simulink model "hyd_hyb_2_int_cont_Final_AMT"  (R2013b)
settings: Solver=ode4  StartTime=0  StopTime=3005  FixedStep=0.01  MaxStep=.4  RelTol=1e-8
InitFcn:
  | const_3_new
values from neighbouring files (symbols this model uses):
  Af = 6.3    [brk_enrg.m]    (also in brk_enrg_1.m)
  BSFC_906_205 = [3.5684 4.3466 5.1668 6.0769 6.988 7.8992 8.8104 9.7336 10.8548 11.9809 13.1112 14.2571 ... (663 elements, 39x17)]    [BSFC_map_906_205.mat]
  Cd = 0.55    [brk_enrg.m]    (also in brk_enrg_1.m)
  den = 1.202    [brk_enrg.m]    (also in brk_enrg_1.m)
  fr = 0.01    [brk_enrg.m]    (also in brk_enrg_1.m)
undefined symbols (not defined in the file or in its folder): clutchRise, down_spd_2, down_spd_3, down_spd_4, down_spd_c, Driving_Cycle, fuel_density, gearshift, I_wheel, Idle_spd_eng_906, M1_hydr, p_v_15, pmax_125, qv_125, Rw, sec_eng_sfc_map, T0, T1, T_max_906, T_min, TC_spd_ratio_max, teta_new_10, torque_convertor, Twait, up_spd_1, up_spd_2, up_spd_3, up_spd_c, v_p_10, v_p_15, v_p_5
libraries: neural x1742, fl_lib x43, nesl_utility x30, sdl_lib x14, simulink x4, simulink_need_slupdate x1
(part 13 of 26)

== system hyd_hyb_2_int_cont_Final_AMT/controller1/optimized controller/SOC upper 0.5/SOC under 0.6/net_loc_rod_5_6/Layer 3/Delays 1 ==
  "p{3}" : Inport  PortDimensions=60
  mux : Mux  Inputs=1
  "pd{3,2}" : Outport
  wires:
  "p{3}"/1 -> mux/1
  mux/1 -> "pd{3,2}"/1

== system hyd_hyb_2_int_cont_Final_AMT/controller1/optimized controller/SOC upper 0.5/SOC under 0.6/net_loc_rod_5_6/Layer 3/LW{3,2} ==
  "ad{3,2}" : Inport  PortDimensions=60
  "IW{3,2}(1,:)'" : Constant  Value=[0.21278300477895107;0.51344852513289463;-0.037590241773840127;0.87426964561402842;0.47883974451806377;-0.50784781099782816;-0.42443313454818898;-0.63652603538509656;0.70423364527984744;0.58568292864178184;-0.52796615746288977;-0.44287483766577246;0.86901354772123618;-0.13831685526252785;0.86566149289060479;0.64403142490178156;0.71733541437838555;0.027462260085903828;-0.37265143230844694;0.71199097292665836;-1.0092668976607591;0.54326870405319294;-0.22161113024701684;0.22850993838939238;-0.056916095287317267;-0.91628445056316477;-0.91086476780370962;-0.060619157895533675;0.93064231354933902;0.57914173943359415;0.22128542734464982;0.7199158978518877;0.9270211186610392;-0.82882792624492585;-0.35445656093166766;0.56586404922693345;0.21840031287896147;0.12031889714860289;0.61358543472489502;-0.34437004445453206;-0.49319773551856233;0.74417786809055086;0.83416465722893218;0.025074562352173025;-0.65605871255971948;-0.98066330920260369;-0.79678322946662417;-0.33944765090641305;-0.80799595485443365;0.73951954905542505;0.90293635064930589;-0.53403515470352247;-0.99336400775468636;0.86698814398730517;-0.5677534071583421;-0.32793471469176605;0.14570127648050649;0.0087963951498697922;-0.6729797739571125;0.31101959537299745]
  Mux : Mux  Inputs=1
  dotprod1 : neural/Weight Functions/dotprod
  "lz{3,2}" : Outport
  wires:
  "IW{3,2}(1,:)'"/1 -> dotprod1/1
  "ad{3,2}"/1 -> dotprod1/2
  dotprod1/1 -> Mux/1
  Mux/1 -> "lz{3,2}"/1

== system hyd_hyb_2_int_cont_Final_AMT/controller1/optimized controller/SOC upper 0.5/SOC upper 0.6/SOC under 0.7/net_col_a_b_6_1/Layer 1 ==
  "p{1}" : Inport  PortDimensions=2
  Delays 1 : Subsystem
  "IW{1,1}" : Subsystem
  "b{1}" : Constant  Value=[5.4291259813067461;4.718478314630234;3.7592821803800116;-3.1787920472608406;2.2590998726780076;1.3899147707624782;0.87327049833135528;-0.021254336575357417;-0.80530109394321947;-1.4715401148994816;2.2200413751043135;3.0289705769041251;3.923020910366191;4.6547090616272833;5.4114556646704166]
  netsum : Sum  Inputs=2  SaturateOnIntegerOverflow=on  InputSameDT=on  OutDataTypeStr=Inherit: Same as first input
  tansig : neural/Transfer Functions/tansig
  "a{1}" : Outport  InitialOutput=[0;0;0;0;0;0;0;0;0;0;0;0;0;0;0]
  wires:
  "p{1}"/1 -> Delays 1/1("p{1}")
  Delays 1/1("pd{1,1}") -> "IW{1,1}"/1("pd{1,1}")
  "IW{1,1}"/1("iz{1,1}") -> netsum/1
  "b{1}"/1 -> netsum/2
  netsum/1 -> tansig/1
  tansig/1 -> "a{1}"/1

== system hyd_hyb_2_int_cont_Final_AMT/controller1/optimized controller/SOC upper 0.5/SOC upper 0.6/SOC under 0.7/net_col_a_b_6_1/Layer 2 ==
  "a{1} " : Inport  PortDimensions=15
  Delays 1 : Subsystem
  "LW{2,1}" : Subsystem
  "b{2}" : Constant  Value=[-1.646349611515898;-1.5096703195224832;1.3949167909537323;1.1533080996131411;0.98809756853578845;-0.68129902029256906;0.56728877028882763;0.46578866737002761;-0.33256964616945445;0.14197265823532756;-0.011470087521661837;0.27403951081779188;0.44394331190764186;0.63896055064956137;0.67829391232291314;0.97113533342800851;-1.1922907318745983;1.2971020916511706;1.529818326598521;1.6930343749454633]
  netsum : Sum  Inputs=2  SaturateOnIntegerOverflow=on  InputSameDT=on  OutDataTypeStr=Inherit: Same as first input
  tansig : neural/Transfer Functions/tansig
  "a{2}" : Outport  InitialOutput=[0;0;0;0;0;0;0;0;0;0;0;0;0;0;0;0;0;0;0;0]
  wires:
  "a{1} "/1 -> Delays 1/1("p{2}")
  Delays 1/1("pd{2,1}") -> "LW{2,1}"/1("ad{2,1}")
  "LW{2,1}"/1("lz{2,1}") -> netsum/1
  "b{2}"/1 -> netsum/2
  netsum/1 -> tansig/1
  tansig/1 -> "a{2}"/1

== system hyd_hyb_2_int_cont_Final_AMT/controller1/optimized controller/SOC upper 0.5/SOC upper 0.6/SOC under 0.7/net_col_a_b_6_1/Layer 3 ==
  "a{2} " : Inport  PortDimensions=20
  Delays 1 : Subsystem
  "LW{3,2}" : Subsystem
  "b{3}" : Constant  Value=0.042619569041635712
  netsum : Sum  Inputs=2  SaturateOnIntegerOverflow=on  InputSameDT=on  OutDataTypeStr=Inherit: Same as first input
  purelin : neural/Transfer Functions/purelin
  "a{3}" : Outport  InitialOutput=0
  wires:
  "a{2} "/1 -> Delays 1/1("p{3}")
  Delays 1/1("pd{3,2}") -> "LW{3,2}"/1("ad{3,2}")
  "LW{3,2}"/1("lz{3,2}") -> netsum/1
  "b{3}"/1 -> netsum/2
  netsum/1 -> purelin/1
  purelin/1 -> "a{3}"/1

== system hyd_hyb_2_int_cont_Final_AMT/controller1/optimized controller/SOC upper 0.5/SOC upper 0.6/SOC under 0.7/net_col_a_b_6_1/Process Input 1 ==
  x : Inport  PortDimensions=2
  fixunknowns : neural/Processing Functions/fixunknowns  inputSize=2  indices=[1 2]
  mapminmax : neural/Processing Functions/mapminmax  xmin=[0.011694642437567444;0.050000000000000003]  xmax=[1;0.94394666666666693]  ymin=-1  ymax=1
  removeconstantrows : neural/Processing Functions/removeconstantrows  inputSize=2  keep=[1 2]
  p : Outport  PortDimensions=2
  wires:
  x/1 -> fixunknowns/1
  fixunknowns/1 -> removeconstantrows/1
  removeconstantrows/1 -> mapminmax/1
  mapminmax/1 -> p/1

== system hyd_hyb_2_int_cont_Final_AMT/controller1/optimized controller/SOC upper 0.5/SOC upper 0.6/SOC under 0.7/net_col_a_b_6_1/Process Output 1 ==
  a : Inport  PortDimensions=1
  mapminmax_reverse : neural/Processing Functions/mapminmax_reverse  xmin=0  xmax=1  ymin=-1  ymax=1
  removeconstantrows_reverse : neural/Processing Functions/removeconstantrows_reverse  inputSize=1  constants=zeros(0,1)  rearrange=1
  y : Outport  PortDimensions=1
  wires:
  a/1 -> mapminmax_reverse/1
  mapminmax_reverse/1 -> removeconstantrows_reverse/1
  removeconstantrows_reverse/1 -> y/1

== system hyd_hyb_2_int_cont_Final_AMT/controller1/optimized controller/SOC upper 0.5/SOC upper 0.6/SOC under 0.7/net_col_a_b_6_7/Layer 1 ==
  "p{1}" : Inport  PortDimensions=2
  Delays 1 : Subsystem
  "IW{1,1}" : Subsystem
  "b{1}" : Constant  Value=[5.4291259813067461;4.718478314630234;3.7592821803800116;-3.1787920472608406;2.2590998726780076;1.3899147707624782;0.87327049833135528;-0.021254336575357417;-0.80530109394321947;-1.4715401148994816;2.2200413751043135;3.0289705769041251;3.923020910366191;4.6547090616272833;5.4114556646704166]
  netsum : Sum  Inputs=2  SaturateOnIntegerOverflow=on  InputSameDT=on  OutDataTypeStr=Inherit: Same as first input
  tansig : neural/Transfer Functions/tansig
  "a{1}" : Outport  InitialOutput=[0;0;0;0;0;0;0;0;0;0;0;0;0;0;0]
  wires:
  tansig/1 -> "a{1}"/1
  netsum/1 -> tansig/1
  "b{1}"/1 -> netsum/2
  "IW{1,1}"/1("iz{1,1}") -> netsum/1
  Delays 1/1("pd{1,1}") -> "IW{1,1}"/1("pd{1,1}")
  "p{1}"/1 -> Delays 1/1("p{1}")

== system hyd_hyb_2_int_cont_Final_AMT/controller1/optimized controller/SOC upper 0.5/SOC upper 0.6/SOC under 0.7/net_col_a_b_6_7/Layer 2 ==
  "a{1} " : Inport  PortDimensions=15
  Delays 1 : Subsystem
  "LW{2,1}" : Subsystem
  "b{2}" : Constant  Value=[-1.646349611515898;-1.5096703195224832;1.3949167909537323;1.1533080996131411;0.98809756853578845;-0.68129902029256906;0.56728877028882763;0.46578866737002761;-0.33256964616945445;0.14197265823532756;-0.011470087521661837;0.27403951081779188;0.44394331190764186;0.63896055064956137;0.67829391232291314;0.97113533342800851;-1.1922907318745983;1.2971020916511706;1.529818326598521;1.6930343749454633]
  netsum : Sum  Inputs=2  SaturateOnIntegerOverflow=on  InputSameDT=on  OutDataTypeStr=Inherit: Same as first input
  tansig : neural/Transfer Functions/tansig
  "a{2}" : Outport  InitialOutput=[0;0;0;0;0;0;0;0;0;0;0;0;0;0;0;0;0;0;0;0]
  wires:
  tansig/1 -> "a{2}"/1
  netsum/1 -> tansig/1
  "b{2}"/1 -> netsum/2
  "LW{2,1}"/1("lz{2,1}") -> netsum/1
  Delays 1/1("pd{2,1}") -> "LW{2,1}"/1("ad{2,1}")
  "a{1} "/1 -> Delays 1/1("p{2}")

== system hyd_hyb_2_int_cont_Final_AMT/controller1/optimized controller/SOC upper 0.5/SOC upper 0.6/SOC under 0.7/net_col_a_b_6_7/Layer 3 ==
  "a{2} " : Inport  PortDimensions=20
  Delays 1 : Subsystem
  "LW{3,2}" : Subsystem
  "b{3}" : Constant  Value=0.042619569041635712
  netsum : Sum  Inputs=2  SaturateOnIntegerOverflow=on  InputSameDT=on  OutDataTypeStr=Inherit: Same as first input
  purelin : neural/Transfer Functions/purelin
  "a{3}" : Outport  InitialOutput=0
  wires:
  purelin/1 -> "a{3}"/1
  netsum/1 -> purelin/1
  "b{3}"/1 -> netsum/2
  "LW{3,2}"/1("lz{3,2}") -> netsum/1
  Delays 1/1("pd{3,2}") -> "LW{3,2}"/1("ad{3,2}")
  "a{2} "/1 -> Delays 1/1("p{3}")

== system hyd_hyb_2_int_cont_Final_AMT/controller1/optimized controller/SOC upper 0.5/SOC upper 0.6/SOC under 0.7/net_col_a_b_6_7/Process Input 1 ==
  x : Inport  PortDimensions=2
  fixunknowns : neural/Processing Functions/fixunknowns  inputSize=2  indices=[1 2]
  mapminmax : neural/Processing Functions/mapminmax  xmin=[0.011694642437567444;0.050000000000000003]  xmax=[1;0.94394666666666693]  ymin=-1  ymax=1
  removeconstantrows : neural/Processing Functions/removeconstantrows  inputSize=2  keep=[1 2]
  p : Outport  PortDimensions=2
  wires:
  mapminmax/1 -> p/1
  removeconstantrows/1 -> mapminmax/1
  fixunknowns/1 -> removeconstantrows/1
  x/1 -> fixunknowns/1

== system hyd_hyb_2_int_cont_Final_AMT/controller1/optimized controller/SOC upper 0.5/SOC upper 0.6/SOC under 0.7/net_col_a_b_6_7/Process Output 1 ==
  a : Inport  PortDimensions=1
  mapminmax_reverse : neural/Processing Functions/mapminmax_reverse  xmin=0  xmax=1  ymin=-1  ymax=1
  removeconstantrows_reverse : neural/Processing Functions/removeconstantrows_reverse  inputSize=1  constants=zeros(0,1)  rearrange=1
  y : Outport  PortDimensions=1
  wires:
  removeconstantrows_reverse/1 -> y/1
  mapminmax_reverse/1 -> removeconstantrows_reverse/1
  a/1 -> mapminmax_reverse/1

== system hyd_hyb_2_int_cont_Final_AMT/controller1/optimized controller/SOC upper 0.5/SOC upper 0.6/SOC under 0.7/net_col_e_f_6_7/Layer 1 ==
  "p{1}" : Inport  PortDimensions=2
  Delays 1 : Subsystem
  "IW{1,1}" : Subsystem
  "b{1}" : Constant  Value=[-8.8578922704763041;8.4042892360625192;-7.9500084893405489;7.492292740917911;-7.075297682831537;6.5653391411727364;6.140320418383804;-5.6306218037143498;5.2017310942740975;4.7779398662401924;-4.3096479437985149;-3.8694939533350459;-3.4026972434889582;2.9180363550485859;2.5233555299387724;2.0614869063433754;1.5965524496681351;-1.1423406487569012;0.64405884107426203;0.23295690475029907;0.21904951735863054;0.68273518079764783;1.1340220880771177;1.4628899047128925;-2.0189679486955385;-2.6776183293763673;2.9490574244714782;3.4373185112780584;3.8603599158778059;4.3183089131402985;-4.7896523588348439;5.2017411095223869;-5.6883600090125501;-6.1259092722430823;6.6028020849475491;7.0422452842927754;-7.4915663488509772;7.9665515781619485;-8.3941668997364953;-8.8548095629012451]
  netsum : Sum  Inputs=2  SaturateOnIntegerOverflow=on  InputSameDT=on  OutDataTypeStr=Inherit: Same as first input
  tansig : neural/Transfer Functions/tansig
  "a{1}" : Outport  InitialOutput=[0;0;0;0;0;0;0;0;0;0;0;0;0;0;0;0;0;0;0;0;0;0;0;0;0;0;0;0;0;0;0;0;0;0;0;0;0;0;0;0]
  wires:
  tansig/1 -> "a{1}"/1
  netsum/1 -> tansig/1
  "b{1}"/1 -> netsum/2
  "IW{1,1}"/1("iz{1,1}") -> netsum/1
  Delays 1/1("pd{1,1}") -> "IW{1,1}"/1("pd{1,1}")
  "p{1}"/1 -> Delays 1/1("p{1}")

== system hyd_hyb_2_int_cont_Final_AMT/controller1/optimized controller/SOC upper 0.5/SOC upper 0.6/SOC under 0.7/net_col_e_f_6_7/Layer 2 ==
  "a{1} " : Inport  PortDimensions=40
  Delays 1 : Subsystem
  "LW{2,1}" : Subsystem
  "b{2}" : Constant  Value=[-1.5481410379896341;-1.4722157754701299;-1.4182962377280097;-1.3387311384343061;1.2983921636824405;-1.210024697487539;1.1647052885200337;1.085322627026474;-1.0583259785438344;-1.0125038796374846;-0.92816237918533084;-0.84166214172462495;0.7720476266891465;-0.68862710060922727;-0.66180234799140847;0.55778737249163612;-0.5739733374634064;-0.45525711092005827;-0.40942953136334892;0.36574767859724377;0.27529894302507696;0.24383222824829606;0.19268525262761244;-0.0869252647609811;-0.040403947124311022;-0.031888545879754718;-0.05798707962786407;0.13694331166074308;0.24631659120042129;0.26591880237517995;0.32068778652282787;0.37526588045543213;-0.47498839316153901;0.51137673885021073;-0.5990164565810322;0.67203954642275587;0.7511674885213897;-0.77140397482380441;0.85976576557099027;-0.92388442298986573;0.96930527326269178;-1.0298098139986036;-1.1007021830056818;1.1648435654146696;1.2287555475076584;-1.2833186739340898;-1.3606363399356558;1.4167612982858691;-1.5157208154592794;1.5087905241510864]
  netsum : Sum  Inputs=2  SaturateOnIntegerOverflow=on  InputSameDT=on  OutDataTypeStr=Inherit: Same as first input
  tansig : neural/Transfer Functions/tansig
  "a{2}" : Outport  InitialOutput=[0;0;0;0;0;0;0;0;0;0;0;0;0;0;0;0;0;0;0;0;0;0;0;0;0;0;0;0;0;0;0;0;0;0;0;0;0;0;0;0;0;0;0;0;0;0;0;0;0;0]
  wires:
  tansig/1 -> "a{2}"/1
  netsum/1 -> tansig/1
  "b{2}"/1 -> netsum/2
  "LW{2,1}"/1("lz{2,1}") -> netsum/1
  Delays 1/1("pd{2,1}") -> "LW{2,1}"/1("ad{2,1}")
  "a{1} "/1 -> Delays 1/1("p{2}")

== system hyd_hyb_2_int_cont_Final_AMT/controller1/optimized controller/SOC upper 0.5/SOC upper 0.6/SOC under 0.7/net_col_e_f_6_7/Layer 3 ==
  "a{2} " : Inport  PortDimensions=50
  Delays 1 : Subsystem
  "LW{3,2}" : Subsystem
  "b{3}" : Constant  Value=-0.11506746394677372
  netsum : Sum  Inputs=2  SaturateOnIntegerOverflow=on  InputSameDT=on  OutDataTypeStr=Inherit: Same as first input
  purelin : neural/Transfer Functions/purelin
  "a{3}" : Outport  InitialOutput=0
  wires:
  purelin/1 -> "a{3}"/1
  netsum/1 -> purelin/1
  "b{3}"/1 -> netsum/2
  "LW{3,2}"/1("lz{3,2}") -> netsum/1
  Delays 1/1("pd{3,2}") -> "LW{3,2}"/1("ad{3,2}")
  "a{2} "/1 -> Delays 1/1("p{3}")

== system hyd_hyb_2_int_cont_Final_AMT/controller1/optimized controller/SOC upper 0.5/SOC upper 0.6/SOC under 0.7/net_col_e_f_6_7/Process Input 1 ==
  x : Inport  PortDimensions=2
  fixunknowns : neural/Processing Functions/fixunknowns  inputSize=2  indices=[1 2]
  mapminmax : neural/Processing Functions/mapminmax  xmin=[0.0027835059349667611;0.021539146666666665]  xmax=[1.009090909090909;0.58889400000000003]  ymin=-1  ymax=1
  removeconstantrows : neural/Processing Functions/removeconstantrows  inputSize=2  keep=[1 2]
  p : Outport  PortDimensions=2
  wires:
  mapminmax/1 -> p/1
  removeconstantrows/1 -> mapminmax/1
  fixunknowns/1 -> removeconstantrows/1
  x/1 -> fixunknowns/1

== system hyd_hyb_2_int_cont_Final_AMT/controller1/optimized controller/SOC upper 0.5/SOC upper 0.6/SOC under 0.7/net_col_e_f_6_7/Process Output 1 ==
  a : Inport  PortDimensions=1
  mapminmax_reverse : neural/Processing Functions/mapminmax_reverse  xmin=0  xmax=1  ymin=-1  ymax=1
  removeconstantrows_reverse : neural/Processing Functions/removeconstantrows_reverse  inputSize=1  constants=zeros(0,1)  rearrange=1
  y : Outport  PortDimensions=1
  wires:
  removeconstantrows_reverse/1 -> y/1
  mapminmax_reverse/1 -> removeconstantrows_reverse/1
  a/1 -> mapminmax_reverse/1

== system hyd_hyb_2_int_cont_Final_AMT/controller1/optimized controller/SOC upper 0.5/SOC upper 0.6/SOC under 0.7/net_loc_rod_6_7/Layer 1 ==
  "p{1}" : Inport  PortDimensions=2
  Delays 1 : Subsystem
  "IW{1,1}" : Subsystem
  "b{1}" : Constant  Value=[8.824474549246748;-8.3539581899361774;7.9180500965715499;7.4856270452295295;7.0291889559197109;-6.5160648504037608;-6.0051491737445231;-5.6799709048951863;5.19806155256191;4.7694002581991688;-4.2718293307910846;-3.7933727449376735;-3.4075974872825943;-2.9557662001981453;-2.4512826171554551;1.9968540619284594;-1.5180712033708814;-1.0823236947351929;0.65270333067677622;-0.22171360341636442;0.30648910984876571;-0.65165847547612499;-1.1471337479688715;1.5911971989977467;-2.0449450710405568;-2.4302538050746536;2.9621146231919044;-3.4741028886743219;3.8037991235467468;4.0802221372092466;-4.6712341146850189;-5.1980673102079908;5.6856540997831884;-6.1501781260260069;6.5094993739119937;-7.0017996579089372;-7.4043669072906422;7.8466649688215488;-8.274364497349513;8.7769344884722695]
  netsum : Sum  Inputs=2  SaturateOnIntegerOverflow=on  InputSameDT=on  OutDataTypeStr=Inherit: Same as first input
  tansig : neural/Transfer Functions/tansig
  "a{1}" : Outport  InitialOutput=[0;0;0;0;0;0;0;0;0;0;0;0;0;0;0;0;0;0;0;0;0;0;0;0;0;0;0;0;0;0;0;0;0;0;0;0;0;0;0;0]
  wires:
  tansig/1 -> "a{1}"/1
  netsum/1 -> tansig/1
  "b{1}"/1 -> netsum/2
  "IW{1,1}"/1("iz{1,1}") -> netsum/1
  Delays 1/1("pd{1,1}") -> "IW{1,1}"/1("pd{1,1}")
  "p{1}"/1 -> Delays 1/1("p{1}")

== system hyd_hyb_2_int_cont_Final_AMT/controller1/optimized controller/SOC upper 0.5/SOC upper 0.6/SOC under 0.7/net_loc_rod_6_7/Layer 2 ==
  "a{1} " : Inport  PortDimensions=40
  Delays 1 : Subsystem
  "LW{2,1}" : Subsystem
  "b{2}" : Constant  Value=[-1.5375109884301688;1.4171736518535769;1.52361155268007;1.3748031344760954;1.3228743192422741;1.2710869402908649;-1.2289478762921457;1.3043666245357657;1.1279084073962473;1.1592324888470029;1.0816615754733507;-1.1076579897629193;-0.91501169053418618;-0.94094658429811684;0.87746244560174713;0.94827946297111543;-0.85279014408642195;-0.55136865473041252;-0.71502898154289862;0.56062094302079912;-0.49981430410271727;0.5080931190367296;0.50678293785240025;-0.43330284501716315;0.24334211509970571;0.21958195465029282;-0.24935850636213924;-0.26038595402420367;0.19673396450795588;0.13998297555788999;-0.12995027624444025;0.073341413956929349;0.020500738682947012;0.10260269951590015;-0.011977356867705572;0.16529983194991943;0.27248116401324118;0.21972273308017506;0.27831436153061456;-0.37368385210235811;-0.35879821627249703;0.44905820177632477;0.4408842695857364;-0.52649284822534737;-0.52055294018007991;0.71915173123359;-0.57712246944047207;-0.639525224204745;0.78332227425292;-0.91876770100677474;0.74496747317097645;0.81162931619236156;-0.86905432344573885;0.94311832117696659;-1.052080950287456;-1.1540738973387714;1.1288625875898872;1.1443800540884874;1.2742597641129052;1.1542657972950399;-1.3842695887293082;1.4535463851249286;1.4217009587894542;-1.4529796844905569;-1.5186643879755066]
  netsum : Sum  Inputs=2  SaturateOnIntegerOverflow=on  InputSameDT=on  OutDataTypeStr=Inherit: Same as first input
  tansig : neural/Transfer Functions/tansig
  "a{2}" : Outport  InitialOutput=[0;0;0;0;0;0;0;0;0;0;0;0;0;0;0;0;0;0;0;0;0;0;0;0;0;0;0;0;0;0;0;0;0;0;0;0;0;0;0;0;0;0;0;0;0;0;0;0;0;0;0;0;0;0;0;0;0;0;0;0;0;0;0;0;0]
  wires:
  tansig/1 -> "a{2}"/1
  netsum/1 -> tansig/1
  "b{2}"/1 -> netsum/2
  "LW{2,1}"/1("lz{2,1}") -> netsum/1
  Delays 1/1("pd{2,1}") -> "LW{2,1}"/1("ad{2,1}")
  "a{1} "/1 -> Delays 1/1("p{2}")

== system hyd_hyb_2_int_cont_Final_AMT/controller1/optimized controller/SOC upper 0.5/SOC upper 0.6/SOC under 0.7/net_loc_rod_6_7/Layer 3 ==
  "a{2} " : Inport  PortDimensions=65
  Delays 1 : Subsystem
  "LW{3,2}" : Subsystem
  "b{3}" : Constant  Value=-0.44014037970907371
  netsum : Sum  Inputs=2  SaturateOnIntegerOverflow=on  InputSameDT=on  OutDataTypeStr=Inherit: Same as first input
  purelin : neural/Transfer Functions/purelin
  "a{3}" : Outport  InitialOutput=0
  wires:
  purelin/1 -> "a{3}"/1
  netsum/1 -> purelin/1
  "b{3}"/1 -> netsum/2
  "LW{3,2}"/1("lz{3,2}") -> netsum/1
  Delays 1/1("pd{3,2}") -> "LW{3,2}"/1("ad{3,2}")
  "a{2} "/1 -> Delays 1/1("p{3}")

== system hyd_hyb_2_int_cont_Final_AMT/controller1/optimized controller/SOC upper 0.5/SOC upper 0.6/SOC under 0.7/net_loc_rod_6_7/Process Input 1 ==
  x : Inport  PortDimensions=2
  fixunknowns : neural/Processing Functions/fixunknowns  inputSize=2  indices=[1 2]
  mapminmax : neural/Processing Functions/mapminmax  xmin=[0.0018488517726022993;0.17698999999999998]  xmax=[1;0.55617766666666668]  ymin=-1  ymax=1
  removeconstantrows : neural/Processing Functions/removeconstantrows  inputSize=2  keep=[1 2]
  p : Outport  PortDimensions=2
  wires:
  mapminmax/1 -> p/1
  removeconstantrows/1 -> mapminmax/1
  fixunknowns/1 -> removeconstantrows/1
  x/1 -> fixunknowns/1

== system hyd_hyb_2_int_cont_Final_AMT/controller1/optimized controller/SOC upper 0.5/SOC upper 0.6/SOC under 0.7/net_loc_rod_6_7/Process Output 1 ==
  a : Inport  PortDimensions=1
  mapminmax_reverse : neural/Processing Functions/mapminmax_reverse  xmin=0  xmax=1  ymin=-1  ymax=1
  removeconstantrows_reverse : neural/Processing Functions/removeconstantrows_reverse  inputSize=1  constants=zeros(0,1)  rearrange=1
  y : Outport  PortDimensions=1
  wires:
  removeconstantrows_reverse/1 -> y/1
  mapminmax_reverse/1 -> removeconstantrows_reverse/1
  a/1 -> mapminmax_reverse/1

== system hyd_hyb_2_int_cont_Final_AMT/controller1/optimized controller/SOC upper 0.5/SOC upper 0.6/SOC upper 0.7/SOC under 0.8/net_col_a_b_7_8 ==
  Input : Inport  PortDimensions=2
  Layer 1 : Subsystem
  Layer 2 : Subsystem
  Layer 3 : Subsystem
  Process Input 1 : Subsystem
  Process Output 1 : Subsystem
  Output : Outport  InitialOutput=0
  wires:
  Layer 3/1("a{3}") -> Process Output 1/1(a)
  [feedback2] -> Layer 3/1("a{2} ")
  Layer 2/1("a{2}") -> [feedback2]
  [feedback1] -> Layer 2/1("a{1} ")
  Layer 1/1("a{1}") -> [feedback1]
  Process Input 1/1(p) -> Layer 1/1("p{1}")
  Process Output 1/1(y) -> Output/1
  Input/1 -> Process Input 1/1(x)

== system hyd_hyb_2_int_cont_Final_AMT/controller1/optimized controller/SOC upper 0.5/SOC upper 0.6/SOC upper 0.7/SOC under 0.8/net_col_c_d_7_8 ==
  Input : Inport  PortDimensions=2
  Layer 1 : Subsystem
  Layer 2 : Subsystem
  Layer 3 : Subsystem
  Process Input 1 : Subsystem
  Process Output 1 : Subsystem
  Output : Outport  InitialOutput=0
  wires:
  Layer 3/1("a{3}") -> Process Output 1/1(a)
  [feedback2] -> Layer 3/1("a{2} ")
  Layer 2/1("a{2}") -> [feedback2]
  [feedback1] -> Layer 2/1("a{1} ")
  Layer 1/1("a{1}") -> [feedback1]
  Process Input 1/1(p) -> Layer 1/1("p{1}")
  Process Output 1/1(y) -> Output/1
  Input/1 -> Process Input 1/1(x)

== system hyd_hyb_2_int_cont_Final_AMT/controller1/optimized controller/SOC upper 0.5/SOC upper 0.6/SOC upper 0.7/SOC under 0.8/net_col_e_f_7_8 ==
  Input : Inport  PortDimensions=2
  Layer 1 : Subsystem
  Layer 2 : Subsystem
  Layer 3 : Subsystem
  Process Input 1 : Subsystem
  Process Output 1 : Subsystem
  Output : Outport  InitialOutput=0
  wires:
  Layer 3/1("a{3}") -> Process Output 1/1(a)
  [feedback2] -> Layer 3/1("a{2} ")
  Layer 2/1("a{2}") -> [feedback2]
  [feedback1] -> Layer 2/1("a{1} ")
  Layer 1/1("a{1}") -> [feedback1]
  Process Input 1/1(p) -> Layer 1/1("p{1}")
  Process Output 1/1(y) -> Output/1
  Input/1 -> Process Input 1/1(x)

== system hyd_hyb_2_int_cont_Final_AMT/controller1/optimized controller/SOC upper 0.5/SOC upper 0.6/SOC upper 0.7/SOC under 0.8/net_loc_rod_7_8 ==
  Input : Inport  PortDimensions=2
  Layer 1 : Subsystem
  Layer 2 : Subsystem
  Layer 3 : Subsystem
  Process Input 1 : Subsystem
  Process Output 1 : Subsystem
  Output : Outport  InitialOutput=0
  wires:
  Layer 3/1("a{3}") -> Process Output 1/1(a)
  [feedback2] -> Layer 3/1("a{2} ")
  Layer 2/1("a{2}") -> [feedback2]
  [feedback1] -> Layer 2/1("a{1} ")
  Layer 1/1("a{1}") -> [feedback1]
  Process Input 1/1(p) -> Layer 1/1("p{1}")
  Process Output 1/1(y) -> Output/1
  Input/1 -> Process Input 1/1(x)

== system hyd_hyb_2_int_cont_Final_AMT/controller1/optimized controller/SOC upper 0.5/SOC upper 0.6/SOC upper 0.7/SOC upper 0.8/net_col_a_b_8_9 ==
  Input : Inport  PortDimensions=2
  Layer 1 : Subsystem
  Layer 2 : Subsystem
  Layer 3 : Subsystem
  Process Input 1 : Subsystem
  Process Output 1 : Subsystem
  Output : Outport  InitialOutput=0
  wires:
  Layer 3/1("a{3}") -> Process Output 1/1(a)
  [feedback2] -> Layer 3/1("a{2} ")
  Layer 2/1("a{2}") -> [feedback2]
  [feedback1] -> Layer 2/1("a{1} ")
  Layer 1/1("a{1}") -> [feedback1]
  Process Input 1/1(p) -> Layer 1/1("p{1}")
  Process Output 1/1(y) -> Output/1
  Input/1 -> Process Input 1/1(x)

== system hyd_hyb_2_int_cont_Final_AMT/controller1/optimized controller/SOC upper 0.5/SOC upper 0.6/SOC upper 0.7/SOC upper 0.8/net_col_c_d_8_9 ==
  Input : Inport  PortDimensions=2
  Layer 1 : Subsystem
  Layer 2 : Subsystem
  Layer 3 : Subsystem
  Process Input 1 : Subsystem
  Process Output 1 : Subsystem
  Output : Outport  InitialOutput=0
  wires:
  Layer 3/1("a{3}") -> Process Output 1/1(a)
  [feedback2] -> Layer 3/1("a{2} ")
  Layer 2/1("a{2}") -> [feedback2]
  [feedback1] -> Layer 2/1("a{1} ")
  Layer 1/1("a{1}") -> [feedback1]
  Process Input 1/1(p) -> Layer 1/1("p{1}")
  Process Output 1/1(y) -> Output/1
  Input/1 -> Process Input 1/1(x)

== system hyd_hyb_2_int_cont_Final_AMT/controller1/optimized controller/SOC upper 0.5/SOC upper 0.6/SOC upper 0.7/SOC upper 0.8/net_col_e_f_8_9 ==
  Input : Inport  PortDimensions=2
  Layer 1 : Subsystem
  Layer 2 : Subsystem
  Layer 3 : Subsystem
  Process Input 1 : Subsystem
  Process Output 1 : Subsystem
  Output : Outport  InitialOutput=0
  wires:
  Layer 3/1("a{3}") -> Process Output 1/1(a)
  [feedback2] -> Layer 3/1("a{2} ")
  Layer 2/1("a{2}") -> [feedback2]
  [feedback1] -> Layer 2/1("a{1} ")
  Layer 1/1("a{1}") -> [feedback1]
  Process Input 1/1(p) -> Layer 1/1("p{1}")
  Process Output 1/1(y) -> Output/1
  Input/1 -> Process Input 1/1(x)

== system hyd_hyb_2_int_cont_Final_AMT/controller1/optimized controller/SOC upper 0.5/SOC upper 0.6/SOC upper 0.7/SOC upper 0.8/net_loc_rod_8_9 ==
  Input : Inport  PortDimensions=2
  Layer 1 : Subsystem
  Layer 2 : Subsystem
  Layer 3 : Subsystem
  Process Input 1 : Subsystem
  Process Output 1 : Subsystem
  Output : Outport  InitialOutput=0
  wires:
  Layer 3/1("a{3}") -> Process Output 1/1(a)
  [feedback2] -> Layer 3/1("a{2} ")
  Layer 2/1("a{2}") -> [feedback2]
  [feedback1] -> Layer 2/1("a{1} ")
  Layer 1/1("a{1}") -> [feedback1]
  Process Input 1/1(p) -> Layer 1/1("p{1}")
  Process Output 1/1(y) -> Output/1
  Input/1 -> Process Input 1/1(x)

== system hyd_hyb_2_int_cont_Final_AMT/controller1/optimized controller/SOC upper 0.5/SOC upper 0.6/SOC under 0.7/net_col_a_b_6_1/Layer 1/Delays 1 ==
  "p{1}" : Inport  PortDimensions=2
  mux : Mux  Inputs=1
  "pd{1,1}" : Outport
  wires:
  "p{1}"/1 -> mux/1
  mux/1 -> "pd{1,1}"/1

== system hyd_hyb_2_int_cont_Final_AMT/controller1/optimized controller/SOC upper 0.5/SOC upper 0.6/SOC under 0.7/net_col_a_b_6_1/Layer 1/IW{1,1} ==
  "pd{1,1}" : Inport  PortDimensions=2
  "IW{1,1}(1,:)'" : Constant  Value=[-2.9215529451269213;-4.5605231901592038]
  "IW{1,1}(10,:)'" : Constant  Value=[-5.3570885750041555;1.0904676184842836]
  "IW{1,1}(11,:)'" : Constant  Value=[0.83824931783313861;-5.4202250643121461]
  "IW{1,1}(12,:)'" : Constant  Value=[1.6421801160932843;5.2025670197089289]
  "IW{1,1}(13,:)'" : Constant  Value=[2.896114368535184;-4.5461436964303523]
  "IW{1,1}(14,:)'" : Constant  Value=[5.3499224216880776;0.78085635209939019]
  "IW{1,1}(15,:)'" : Constant  Value=[3.3008677310781862;4.3128757959876163]
  "IW{1,1}(2,:)'" : Constant  Value=[-2.8586637641315789;-4.5350950146401168]
  "IW{1,1}(3,:)'" : Constant  Value=[-3.6697545499151838;4.0894109492261554]
  "IW{1,1}(4,:)'" : Constant  Value=[2.947899693841062;4.5281254034159817]
  "IW{1,1}(5,:)'" : Constant  Value=[-5.0022481161267578;-2.1558205159532036]
  "IW{1,1}(6,:)'" : Constant  Value=[-5.4734688498154087;-0.084237551137234773]
  "IW{1,1}(7,:)'" : Constant  Value=[-2.818576936167271;4.6179415818267469]
  "IW{1,1}(8,:)'" : Constant  Value=[0.95149799776462995;5.3489766501190106]
  "IW{1,1}(9,:)'" : Constant  Value=[-3.6203669694216494;-4.096644931500844]
  Mux : Mux  Inputs=15
  dotprod{1..15} (15 alike) : neural/Weight Functions/dotprod
  "iz{1,1}" : Outport
  wires:
  "IW{1,1}(1,:)'"/1 -> dotprod1/1
  "pd{1,1}"/1 -> dotprod1/2, dotprod2/2, dotprod3/2, dotprod4/2, dotprod5/2, dotprod6/2, dotprod7/2, dotprod8/2, dotprod9/2, dotprod10/2, dotprod11/2, dotprod12/2, dotprod13/2, dotprod14/2, dotprod15/2
  dotprod1/1 -> Mux/1
  "IW{1,1}(2,:)'"/1 -> dotprod2/1
  dotprod2/1 -> Mux/2
  "IW{1,1}(3,:)'"/1 -> dotprod3/1
  dotprod3/1 -> Mux/3
  "IW{1,1}(4,:)'"/1 -> dotprod4/1
  dotprod4/1 -> Mux/4
  "IW{1,1}(5,:)'"/1 -> dotprod5/1
  dotprod5/1 -> Mux/5
  "IW{1,1}(6,:)'"/1 -> dotprod6/1
  dotprod6/1 -> Mux/6
  "IW{1,1}(7,:)'"/1 -> dotprod7/1
  dotprod7/1 -> Mux/7
  "IW{1,1}(8,:)'"/1 -> dotprod8/1
  dotprod8/1 -> Mux/8
  "IW{1,1}(9,:)'"/1 -> dotprod9/1
  dotprod9/1 -> Mux/9
  "IW{1,1}(10,:)'"/1 -> dotprod10/1
  dotprod10/1 -> Mux/10
  "IW{1,1}(11,:)'"/1 -> dotprod11/1
  dotprod11/1 -> Mux/11
  "IW{1,1}(12,:)'"/1 -> dotprod12/1
  dotprod12/1 -> Mux/12
  "IW{1,1}(13,:)'"/1 -> dotprod13/1
  dotprod13/1 -> Mux/13
  "IW{1,1}(14,:)'"/1 -> dotprod14/1
  dotprod14/1 -> Mux/14
  "IW{1,1}(15,:)'"/1 -> dotprod15/1
  dotprod15/1 -> Mux/15
  Mux/1 -> "iz{1,1}"/1

== system hyd_hyb_2_int_cont_Final_AMT/controller1/optimized controller/SOC upper 0.5/SOC upper 0.6/SOC under 0.7/net_col_a_b_6_1/Layer 2/Delays 1 ==
  "p{2}" : Inport  PortDimensions=15
  mux : Mux  Inputs=1
  "pd{2,1}" : Outport
  wires:
  "p{2}"/1 -> mux/1
  mux/1 -> "pd{2,1}"/1

== system hyd_hyb_2_int_cont_Final_AMT/controller1/optimized controller/SOC upper 0.5/SOC upper 0.6/SOC under 0.7/net_col_a_b_6_1/Layer 2/LW{2,1} ==
  "ad{2,1}" : Inport  PortDimensions=15
  "IW{2,1}(1,:)'" : Constant  Value=[0.78053014166343337;0.29204864759646343;0.60078593871991481;0.19930621440626281;-0.6417603988784718;0.33501662440183899;-0.039320692942124112;-0.17818770289629898;0.070466356241360939;-0.66502927238801224;-0.32842903100439153;0.20158473933058277;-0.60401576805008483;0.63057683991132762;0.46880386290573689]
  "IW{2,1}(10,:)'" : Constant  Value=[-0.30542783009719876;-0.066026211922728451;-0.35100377549008915;-0.6458951406528961;0.6850695817633381;0.050282872485727714;-0.44195196962407135;-0.71948403799261362;0.4935632179122752;0.200989642702293;-0.64740412469558006;-0.30623454495757785;-0.13820376368835832;0.62066412214227229;0.17661621326669177]
  "IW{2,1}(11,:)'" : Constant  Value=[0.55562311688590493;0.29292130824353235;-0.24419391791645448;0.076845837964054267;0.60243335325886216;0.80506769153284086;-0.62258315480057702;-0.70181319186512137;0.60049372064453754;-0.12668155594586542;0.2553065093083014;-0.018042964286782859;0.4246140714880226;0.28651937946006795;-0.68228531233739165]
  "IW{2,1}(12,:)'" : Constant  Value=[0.44416805338287024;-0.41349849912235709;-0.2531242786660311;0.53251183022901805;-0.32829808880094952;-0.051197223412570408;0.27404319415393802;0.1490633159542053;-0.54269341475467026;0.5760741998500214;-0.0089493484532183008;-0.59671259088667472;-0.47994730366761462;0.71734359409363657;-0.30739574144086385]
  "IW{2,1}(13,:)'" : Constant  Value=[0.15982120682309786;-0.53065964935234877;0.20469363114772193;-0.72220585278335447;0.25545679685766259;0.46446907755731137;-0.73279447878498261;0.33655378845066519;0.61218591810154344;0.32806776740226229;-0.40812289383238065;-0.53302040536360651;0.38560033802278365;-0.11260146758867617;-0.18156471207988037]
  "IW{2,1}(14,:)'" : Constant  Value=[0.45939822916667666;-0.10380478907464295;0.87572221134442962;0.55983631125429267;-0.6443085799942323;-0.438658480407774;0.1355138270898946;0.36487304620458905;0.16874931498791979;-0.61715910709633148;0.036742549389975593;0.57010417817567027;0.25068623188517275;0.21237791145242596;-0.39946964234245058]
  "IW{2,1}(15,:)'" : Constant  Value=[0.47915172534700973;0.27255790315287942;0.22442881940530401;0.7046931447803112;-0.42347258475423294;0.20776969353826535;-0.0029235768347837467;0.54017509885430626;0.3689196436222304;-0.34046687310245394;-0.30779540105947106;0.095620590251799184;-0.71005195669820909;0.14618524222178611;-0.67403650577607799]
  "IW{2,1}(16,:)'" : Constant  Value=[0.17904077524511536;-0.24759703073580216;0.15354503510687395;0.29995487676372212;-0.83029993499257815;-0.54876470636749908;0.1205063780077144;0.21307832098136134;-0.35023088138505193;0.63285269778590514;-0.36348606773018222;0.12068316900064874;-0.58955228467198162;-0.79539775287905845;-0.48918703494261001]
  "IW{2,1}(17,:)'" : Constant  Value=[-0.34794065988557443;0.55219523589663044;0.5143001603488625;-0.22641708498023344;0.50619738437069095;-0.43357233865330164;-0.31471975107068806;0.44989222134038892;0.020171528379251125;-0.49879442794679685;0.69495060944475706;0.18416728478369501;-0.64194628926812813;-0.44892717349124922;-0.02992035603949263]
  "IW{2,1}(18,:)'" : Constant  Value=[0.30331895611664617;-0.12851315036563801;-0.53462584873971397;-0.46371560949317192;0.13988007049048459;-0.40859791032484338;-0.79681484818945858;-0.016377073182308237;-0.38358662973594859;0.35861055563777722;-0.6496507650902974;-0.62090439723521351;0.076840851410475489;0.63048254223125022;-0.17904919957529017]
  "IW{2,1}(19,:)'" : Constant  Value=[0.42136534934876768;-0.094259274675504004;0.38571921238709894;-0.25975786849453808;0.27980642914644399;0.25103986804488559;-0.60536259986501006;-0.77907072761843155;0.36344966644543175;0.37496372736772582;0.21893946612478141;-0.36281736420872207;-0.12483282318384557;0.44599078258141628;0.85808382076373013]
  "IW{2,1}(2,:)'" : Constant  Value=[0.17575627492329865;0.64661608900825296;0.42137302105518887;-0.44175042575697759;-0.4997020622910609;-0.24150363000577296;-0.54227929869906655;-0.030900429610183539;-0.89489142801219335;-0.63703091125729705;0.42177423558752708;0.27215046474187243;-0.34698223791053751;0.66722016984498034;-0.0061883428480007099]
  "IW{2,1}(20,:)'" : Constant  Value=[0.63439636960799195;-0.0079849099056435568;-0.29312179824428075;-0.11661323059913765;-0.059062754602998473;0.42181160788884509;-0.354936423434419;-0.79002736369917981;0.68314796367141561;-0.31626111931508516;0.18488824411974616;-0.62932262549817952;-0.0026698991954153626;0.65819654748933976;0.29779376842812089]
  "IW{2,1}(3,:)'" : Constant  Value=[-0.12217583136931578;-0.63766103817813291;0.43517835173933522;0.63293446833365052;-0.52860303763913297;-0.76213283901609874;0.14191460170451217;-0.11103439622102566;0.73461022496268757;-0.0047405745337899272;-0.009656240798445315;0.37011754169114702;0.47350620034919455;-0.46645161835048304;0.43334555205260494]
  "IW{2,1}(4,:)'" : Constant  Value=[-0.2005453869405778;0.64893992256903765;0.70402350909180733;0.35856884485351742;0.18900524632612653;0.28089732179910709;0.021155364578440541;0.01900818391730108;0.61684363687319277;-0.22545734121955546;-0.77847633978361408;0.5923575841709301;-0.35224507873924205;0.42076565418116368;0.18895037854545177]
  "IW{2,1}(5,:)'" : Constant  Value=[-0.5873832365212881;0.5870340061374888;0.51879881610097367;0.20306262712379949;0.58198472367706588;-0.088541754224339103;0.60265415473813688;-0.49303371593315082;-0.49232604461319407;-0.15524092257009237;-0.059729873946896203;-0.59340865182430658;0.38715282547449376;0.12736848545340604;-0.43961102624085946]
  "IW{2,1}(6,:)'" : Constant  Value=[0.13736446076866377;0.47148069258784503;-0.35630029659432555;-0.48574242196604062;0.69829640255595016;0.74119954705384339;0.70446786249556448;-0.54164780220432129;0.027062046923033337;-0.32813978317482456;0.20312485406186492;0.20471190638401837;-0.27774373666160662;-0.29877561054994162;0.68667414286446171]
  "IW{2,1}(7,:)'" : Constant  Value=[-0.57571717755453788;-0.0059675488607752293;0.66823977219967612;-0.13032210666990385;-0.39771462827240905;0.70065202775840507;0.24651655595225383;0.15421059694834863;-0.45372541376902564;0.45027176851886697;0.26911175175141044;0.66136745379510065;0.46051315523515801;0.44007352575074449;0.3291262643302636]
  "IW{2,1}(8,:)'" : Constant  Value=[-0.13468571110448263;-0.72001015586532779;0.83168168898079686;0.051300439567951731;-0.29413778931308698;0.35588121434291087;0.13832855947874259;-0.52825182599939458;-0.22776972548979266;0.095012379619955262;-0.64412283600444264;0.033898997348194994;0.65343908042137089;0.36369099742500133;-0.11910178969771282]
  "IW{2,1}(9,:)'" : Constant  Value=[0.26997185648634625;0.26405799369778199;-0.37801464377310512;0.68067072958776387;0.63431596479861185;0.21053904943579516;0.50234312720935115;-0.55377188611462114;-0.46914553861348829;-0.55620160039681665;0.020771550954338174;0.29202998467294183;-0.31675450684928891;0.58500586597730353;0.44301086121313571]
  Mux : Mux  Inputs=20
  dotprod{1..20} (20 alike) : neural/Weight Functions/dotprod
  "lz{2,1}" : Outport
  wires:
  "IW{2,1}(1,:)'"/1 -> dotprod1/1
  "ad{2,1}"/1 -> dotprod1/2, dotprod2/2, dotprod3/2, dotprod4/2, dotprod5/2, dotprod6/2, dotprod7/2, dotprod8/2, dotprod9/2, dotprod10/2, dotprod11/2, dotprod12/2, dotprod13/2, dotprod14/2, dotprod15/2, dotprod16/2, dotprod17/2, dotprod18/2, dotprod19/2, dotprod20/2
  dotprod1/1 -> Mux/1
  "IW{2,1}(2,:)'"/1 -> dotprod2/1
  dotprod2/1 -> Mux/2
  "IW{2,1}(3,:)'"/1 -> dotprod3/1
  dotprod3/1 -> Mux/3
  "IW{2,1}(4,:)'"/1 -> dotprod4/1
  dotprod4/1 -> Mux/4
  "IW{2,1}(5,:)'"/1 -> dotprod5/1
  dotprod5/1 -> Mux/5
  "IW{2,1}(6,:)'"/1 -> dotprod6/1
  dotprod6/1 -> Mux/6
  "IW{2,1}(7,:)'"/1 -> dotprod7/1
  dotprod7/1 -> Mux/7
  "IW{2,1}(8,:)'"/1 -> dotprod8/1
  dotprod8/1 -> Mux/8
  "IW{2,1}(9,:)'"/1 -> dotprod9/1
  dotprod9/1 -> Mux/9
  "IW{2,1}(10,:)'"/1 -> dotprod10/1
  dotprod10/1 -> Mux/10
  "IW{2,1}(11,:)'"/1 -> dotprod11/1
  dotprod11/1 -> Mux/11
  "IW{2,1}(12,:)'"/1 -> dotprod12/1
  dotprod12/1 -> Mux/12
  "IW{2,1}(13,:)'"/1 -> dotprod13/1
  dotprod13/1 -> Mux/13
  "IW{2,1}(14,:)'"/1 -> dotprod14/1
  dotprod14/1 -> Mux/14
  "IW{2,1}(15,:)'"/1 -> dotprod15/1
  dotprod15/1 -> Mux/15
  "IW{2,1}(16,:)'"/1 -> dotprod16/1
  dotprod16/1 -> Mux/16
  "IW{2,1}(17,:)'"/1 -> dotprod17/1
  dotprod17/1 -> Mux/17
  "IW{2,1}(18,:)'"/1 -> dotprod18/1
  dotprod18/1 -> Mux/18
  "IW{2,1}(19,:)'"/1 -> dotprod19/1
  dotprod19/1 -> Mux/19
  "IW{2,1}(20,:)'"/1 -> dotprod20/1
  dotprod20/1 -> Mux/20
  Mux/1 -> "lz{2,1}"/1

== system hyd_hyb_2_int_cont_Final_AMT/controller1/optimized controller/SOC upper 0.5/SOC upper 0.6/SOC under 0.7/net_col_a_b_6_1/Layer 3/Delays 1 ==
  "p{3}" : Inport  PortDimensions=20
  mux : Mux  Inputs=1
  "pd{3,2}" : Outport
  wires:
  "p{3}"/1 -> mux/1
  mux/1 -> "pd{3,2}"/1

== system hyd_hyb_2_int_cont_Final_AMT/controller1/optimized controller/SOC upper 0.5/SOC upper 0.6/SOC under 0.7/net_col_a_b_6_1/Layer 3/LW{3,2} ==
  "ad{3,2}" : Inport  PortDimensions=20
  "IW{3,2}(1,:)'" : Constant  Value=[-0.34903886609399382;1.06705366788284;-0.63069522814965984;0.43720033513892198;-0.11763112400213262;-0.71855053606900632;-0.34692052449521499;-0.46231517262753691;1.0151944900739838;-0.45066968253451173;1.1029155009020308;-0.37855254899971402;0.025219381776951783;-0.56955532675060594;0.74416374807652608;0.63806693225984767;-0.10748465748831162;-0.72740367544789852;0.024756316136680077;0.39060697940746125]
  Mux : Mux  Inputs=1
  dotprod1 : neural/Weight Functions/dotprod
  "lz{3,2}" : Outport
  wires:
  "IW{3,2}(1,:)'"/1 -> dotprod1/1
  "ad{3,2}"/1 -> dotprod1/2
  dotprod1/1 -> Mux/1
  Mux/1 -> "lz{3,2}"/1

== system hyd_hyb_2_int_cont_Final_AMT/controller1/optimized controller/SOC upper 0.5/SOC upper 0.6/SOC under 0.7/net_col_a_b_6_7/Layer 1/Delays 1 ==
  "p{1}" : Inport  PortDimensions=2
  mux : Mux  Inputs=1
  "pd{1,1}" : Outport
  wires:
  mux/1 -> "pd{1,1}"/1
  "p{1}"/1 -> mux/1

== system hyd_hyb_2_int_cont_Final_AMT/controller1/optimized controller/SOC upper 0.5/SOC upper 0.6/SOC under 0.7/net_col_a_b_6_7/Layer 1/IW{1,1} ==
  "pd{1,1}" : Inport  PortDimensions=2
  "IW{1,1}(1,:)'" : Constant  Value=[-2.9215529451269213;-4.5605231901592038]
  "IW{1,1}(10,:)'" : Constant  Value=[-5.3570885750041555;1.0904676184842836]
  "IW{1,1}(11,:)'" : Constant  Value=[0.83824931783313861;-5.4202250643121461]
  "IW{1,1}(12,:)'" : Constant  Value=[1.6421801160932843;5.2025670197089289]
  "IW{1,1}(13,:)'" : Constant  Value=[2.896114368535184;-4.5461436964303523]
  "IW{1,1}(14,:)'" : Constant  Value=[5.3499224216880776;0.78085635209939019]
  "IW{1,1}(15,:)'" : Constant  Value=[3.3008677310781862;4.3128757959876163]
  "IW{1,1}(2,:)'" : Constant  Value=[-2.8586637641315789;-4.5350950146401168]
  "IW{1,1}(3,:)'" : Constant  Value=[-3.6697545499151838;4.0894109492261554]
  "IW{1,1}(4,:)'" : Constant  Value=[2.947899693841062;4.5281254034159817]
  "IW{1,1}(5,:)'" : Constant  Value=[-5.0022481161267578;-2.1558205159532036]
  "IW{1,1}(6,:)'" : Constant  Value=[-5.4734688498154087;-0.084237551137234773]
  "IW{1,1}(7,:)'" : Constant  Value=[-2.818576936167271;4.6179415818267469]
  "IW{1,1}(8,:)'" : Constant  Value=[0.95149799776462995;5.3489766501190106]
  "IW{1,1}(9,:)'" : Constant  Value=[-3.6203669694216494;-4.096644931500844]
  Mux : Mux  Inputs=15
  dotprod{1..15} (15 alike) : neural/Weight Functions/dotprod
  "iz{1,1}" : Outport
  wires:
  Mux/1 -> "iz{1,1}"/1
  dotprod15/1 -> Mux/15
  "IW{1,1}(15,:)'"/1 -> dotprod15/1
  dotprod14/1 -> Mux/14
  "IW{1,1}(14,:)'"/1 -> dotprod14/1
  dotprod13/1 -> Mux/13
  "IW{1,1}(13,:)'"/1 -> dotprod13/1
  dotprod12/1 -> Mux/12
  "IW{1,1}(12,:)'"/1 -> dotprod12/1
  dotprod11/1 -> Mux/11
  "IW{1,1}(11,:)'"/1 -> dotprod11/1
  dotprod10/1 -> Mux/10
  "IW{1,1}(10,:)'"/1 -> dotprod10/1
  dotprod9/1 -> Mux/9
  "IW{1,1}(9,:)'"/1 -> dotprod9/1
  dotprod8/1 -> Mux/8
  "IW{1,1}(8,:)'"/1 -> dotprod8/1
  dotprod7/1 -> Mux/7
  "IW{1,1}(7,:)'"/1 -> dotprod7/1
  dotprod6/1 -> Mux/6
  "IW{1,1}(6,:)'"/1 -> dotprod6/1
  dotprod5/1 -> Mux/5
  "IW{1,1}(5,:)'"/1 -> dotprod5/1
  dotprod4/1 -> Mux/4
  "IW{1,1}(4,:)'"/1 -> dotprod4/1
  dotprod3/1 -> Mux/3
  "IW{1,1}(3,:)'"/1 -> dotprod3/1
  dotprod2/1 -> Mux/2
  "IW{1,1}(2,:)'"/1 -> dotprod2/1
  dotprod1/1 -> Mux/1
  "pd{1,1}"/1 -> dotprod15/2, dotprod14/2, dotprod13/2, dotprod12/2, dotprod11/2, dotprod10/2, dotprod9/2, dotprod8/2, dotprod7/2, dotprod6/2, dotprod5/2, dotprod4/2, dotprod3/2, dotprod2/2, dotprod1/2
  "IW{1,1}(1,:)'"/1 -> dotprod1/1

== system hyd_hyb_2_int_cont_Final_AMT/controller1/optimized controller/SOC upper 0.5/SOC upper 0.6/SOC under 0.7/net_col_a_b_6_7/Layer 2/Delays 1 ==
  "p{2}" : Inport  PortDimensions=15
  mux : Mux  Inputs=1
  "pd{2,1}" : Outport
  wires:
  mux/1 -> "pd{2,1}"/1
  "p{2}"/1 -> mux/1
